simulink model "comparisonSIM"  (R2023b)
settings: Solver=VariableStepAuto  StartTime=0.0  StopTime=50  RelTol=1e-3
libraries: mssSimulink x1
settings Model: Creator=arnaud  LastModifiedBy=isido

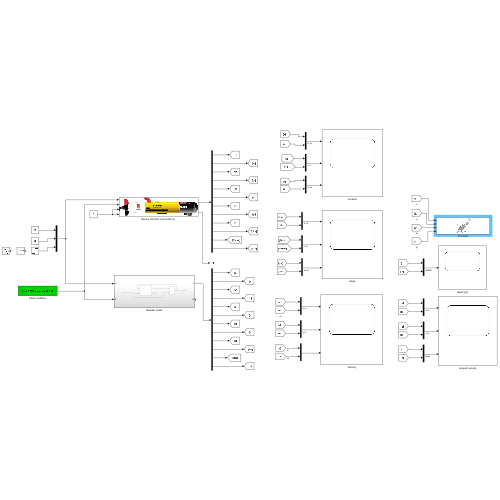
[thumbnail: Simulink's stored preview of the top-level diagram]
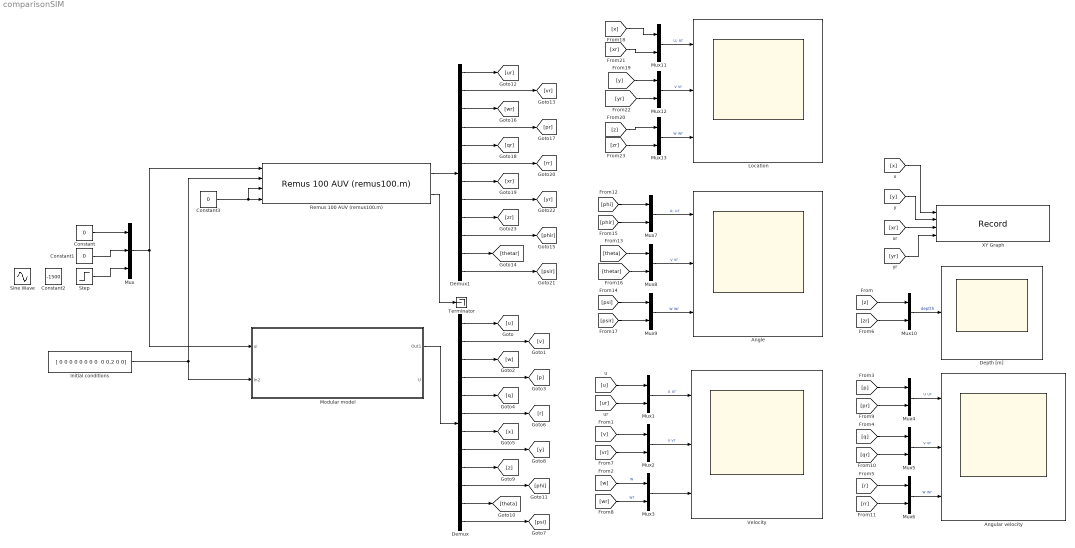
== system comparisonSIM ==
  Angle : Scope  NumInputPorts=3
  Angular velocity : Scope  NumInputPorts=3
  Constant : Constant  Value=0
  Constant1 : Constant  Value=0
  Constant2 : Constant  Value=-1500
  Constant3 : Constant  Value=0
  Demux : Demux  Outputs=12
  Demux1 : Demux  Outputs=12
  Depth [m] : Scope
  Initial conditions : Constant  Value="[ 0 0 0 0 0 0 0 0  0 0.2 0 0]"
  Location : Scope  NumInputPorts=3
  Modular model : Subsystem
  Mux : Mux  Inputs=3
  Mux{1..13} (13 alike) : Mux  Inputs=2
  "Remus 100 AUV (remus100.m) " : mssSimulink/Marine craft models/Remus 100 AUV (remus100.m)  SystemSampleTime=-1  VariantActivationTime=update diagram  AllowFlexibleInterface=on  Latency=0  AutoFrameSizeCalculation=off
  Sine Wave : Sin  Amplitude=1500  SampleTime=0
  Step : Step  Time=2  After=0  SampleTime=0
  Terminator : Terminator
  Velocity : Scope  NumInputPorts=3
  XY Graph : Record  FileSettingsInternal="{\"entries\":[{\"content\":{\"excelSettings\":{\"content\":{},\"type\":\"Streamout.ExcelSettings\"}},\"type\":\"Streamout.FileSettingStorage\",\"uuid\":\"\"}],\"packageUris\":[\"http:\\/\\/schema.mathworks.com\\/mf0\\/streamout_blocks\\/R2020a\"],\"version\":\"1.0\"}"  Layout=[1 1]  SignalsInternal="{\"entries\":[{\"content\":{\"signals\":[{\"content\":{\"blockPath\":[],\"dimensions\":[1],\"domain\":\"\",\"lineColor\":\"#a2142f\",\"plots\":[1],\"port\":1,\"sid\":[\"\"],\"signalID\":9038,\"signalName\":\"x\"},\"type\":\"RecordBlkView.Signal\",\"uuid\":\"\"},{\"content\":{\"blockPath\":[],\"dimensions\":[1],\"domain\":\"\",\"lineColor\":\"#139fff\",\"plots\":[1],\"port\":2,\"sid\":[\"\"],\"signalID\":9042,\"signalName\":\"y\"},\"type\":\"RecordBlkView.Signal\",\"uuid\":\"\"},{\"content\":{\"blockPath\":[],\"dimensions\":[1],\"domain\":\"\",\"lineColor\":\"#edb120\",\"plots\":[1],\"port\":3,\"sid\":[\"\"],\"signalID\":9046,\"signalName\":\"xr\"},\"type\":\"RecordBlkView.Signal\",\"uuid\":\"\"},{\"content\":{\"blockPath\":[],\"dimensions\":[1],\"domain\":\"\",\"lineColor\":\"#7e2f8e\",\"plots\":[1],\"port\":4,\"sid\":[\"\"],\"signalID\":9050,\"signalName\":\"yr\"},\"type\":\"RecordBlkView.Signal\",\"uuid\":\"\"}]},\"type\":\"RecordBlkView.InputSignals\",\"uuid\":\"\"}],\"packageUris\":[\"http:\\/\\/schema.mathworks.com\\/mf0\\/streamout_blocks\\/R2020a\"],\"version\":\"1.0\"}"  VisualizationBindings="{\"xyplotplugin\":{\"info\":[{\"series\":[{\"bindingParametersList\":[{\"parameter\":\"X-Axis\",\"signalID\":9046,\"signalName\":\"xr\"},{\"parameter\":\"Y-Axis\",\"signalID\":9050,\"signalName\":\"yr\"}],\"seriesID\":47107},{\"bindingParametersList\":[{\"parameter\":\"X-Axis\",\"signalID\":9038,\"signalName\":\"x\"},{\"parameter\":\"Y-Axis\",\"signalID\":9042,\"signalName\":\"y\"}],\"seriesID\":22373}],\"subplotID\":1}]}}"  CompatibilityTag=XY
  wires:
  Demux/9 -> [z]
  Demux/8 -> [y]
  Demux/5 -> [q]
  Mux4/1 -> Angular velocity/1  "u ur"
  [wr] -> Mux3/2  "wr"
  [w] -> Mux3/1  "w"
  Mux3/1 -> Velocity/3
  [phi] -> Mux7/1
  [ur] -> Mux1/2
  [thetar] -> Mux8/2
  [psir] -> Mux9/2
  [vr] -> Mux2/2
  [psi] -> Mux9/1
  Demux/3 -> [w]
  [q] -> Mux5/1
  [z] -> Mux10/1
  [x] -> XY Graph/1
  [theta] -> Mux8/1
  [zr] -> Mux10/2
  [phir] -> Mux7/2
  Demux/2 -> [v]
  [y] -> XY Graph/2
  Demux1/5 -> [qr]
  [pr] -> Mux4/2
  Mux8/1 -> Angle/2  "v vr"
  Mux2/1 -> Velocity/2  "v vr"
  Demux/4 -> [p]
  [qr] -> Mux5/2
  Demux1/4 -> [pr]
  [v] -> Mux2/1
  [p] -> Mux4/1
  Demux1/12 -> [psir]
  Mux7/1 -> Angle/1  "u; ur"
  [u] -> Mux1/1
  [yr] -> XY Graph/4
  [xr] -> XY Graph/3
  Constant/1 -> Mux/1
  Mux9/1 -> Angle/3  "w wr"
  Mux6/1 -> Angular velocity/3  "w wr"
  [r] -> Mux6/1
  Mux/1 -> Modular model/1(ui), "Remus 100 AUV (remus100.m) "/1
  Demux/7 -> [x]
  Constant3/1 -> "Remus 100 AUV (remus100.m) "/3, "Remus 100 AUV (remus100.m) "/4
  Initial conditions/1 -> Modular model/2(In2), "Remus 100 AUV (remus100.m) "/2
  Mux1/1 -> Velocity/1  "u ur"
  Demux1/1 -> [ur]
  "Remus 100 AUV (remus100.m) "/1 -> Demux1/1
  "Remus 100 AUV (remus100.m) "/2 -> Terminator/1
  Modular model/1(Out1) -> Demux/1
  Demux/11 -> [theta]
  Demux/10 -> [phi]
  Demux/6 -> [r]
  Demux1/2 -> [vr]
  Demux1/8 -> [yr]
  Demux1/3 -> [wr]
  Mux5/1 -> Angular velocity/2  "v vr"
  Demux1/6 -> [rr]
  [rr] -> Mux6/2
  Demux1/7 -> [xr]
  Demux/12 -> [psi]
  Demux1/9 -> [zr]
  Mux10/1 -> Depth [m]/1  "deptth"
  Demux1/10 -> [phir]
  Demux1/11 -> [thetar]
  Constant1/1 -> Mux/2
  Demux/1 -> [u]
  [y] -> Mux12/1
  [z] -> Mux13/1
  [xr] -> Mux11/2
  [zr] -> Mux13/2
  [yr] -> Mux12/2
  [x] -> Mux11/1
  Mux12/1 -> Location/2  "v vr"
  Mux13/1 -> Location/3  "w wr"
  Mux11/1 -> Location/1  "u; ur"
  Step/1 -> Mux/3

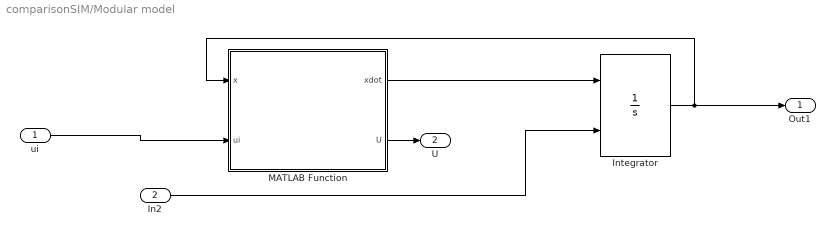
== system comparisonSIM/Modular model ==
  ui : Inport
  In2 : Inport  Port=2
  Integrator : Integrator  InitialConditionSource=external  InitialCondition=zeros(1,12)'
  MATLAB Function : MATLAB Function  TreatAsAtomicUnit=on
  Out1 : Outport
  U : Outport  Port=2
  wires:
  MATLAB Function/1(xdot) -> Integrator/1
  ui/1 -> MATLAB Function/2(ui)
  In2/1 -> Integrator/2
  Integrator/1 -> Out1/1, MATLAB Function/1(x)
  MATLAB Function/2(U) -> U/1

== matlab function comparisonSIM/Modular model/MATLAB Function ==
  data: x input; xdot output size=12; ui input; U output
function [xdot,U] = fcn(x,ui)

[xdot,U] = main_Modular(x,ui);
